simulink model "sandbox_varying"  (R2018b)
settings: Solver=VariableStepAuto  StartTime=0.0  StopTime=20  MaxStep=5e-2  RelTol=1e-3
values from neighbouring files (symbols this model uses):
  B = eye(6)    [eq_setup.m]
  G = [0, 0, m*g, 0, 0, 0]'    [eq_setup.m]
  K_E = 0.05    [eq_setup.m]
  K_m = [[ m*eye(3), zeros(3)] ... (first row only)    [eq_setup.m]
  K_p = [[  K_pt,    zeros(3)] ... (first row only)    [eq_setup.m]
  K_v = [[  K_vt,    zeros(3)] ... (first row only)    [eq_setup.m]
  M = [[ m*eye(3), zeros(3)] ... (first row only)    [eq_setup.m]
  M_inv = inv(M)    [eq_setup.m]
  xi_0 = [p_0, theta_0]    [eq_setup.m]
libraries: simulink x1
settings Model: Creator=valeriiche  LastModifiedBy=valeriiche

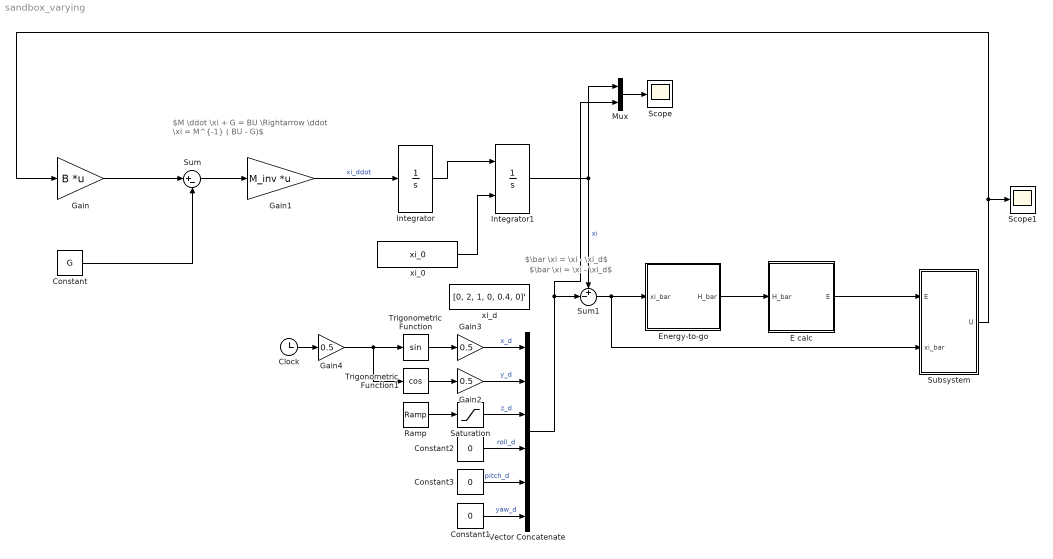
== system sandbox_varying ==
  note: $M \ddot \xi + G = BU \Rightarrow \ddot \xi = M^{-1} ( BU - G)$
  note: $\bar \xi = \xi - \xi_d$
  note: $\bar \xi = \xi - \xi_d$
  Clock : Clock
  Constant : Constant  Value=G
  Constant1 : Constant  Value=0
  Constant2 : Constant  Value=0
  Constant3 : Constant  Value=0
  E calc : Subsystem
  Energy-to-go : Subsystem
  Gain : Gain  Gain=B  Multiplication=Matrix(K*u) (u vector)
  Gain1 : Gain  Gain=M_inv  Multiplication=Matrix(K*u) (u vector)
  Gain2 : Gain  Gain=0.5
  Gain3 : Gain  Gain=0.5
  Gain4 : Gain  Gain=0.5
  Integrator : Integrator
  Integrator1 : Integrator  InitialConditionSource=external
  Mux : Mux  Inputs=2
  Ramp : simulink/Sources/Ramp  slope=0.333  start=0  InitialOutput=0
  Saturation : Saturate  UpperLimit=2  LowerLimit=0
  Scope : Scope
  Scope1 : Scope
  Subsystem : Subsystem
  Sum : Sum  Inputs=|+-
  Sum1 : Sum  Inputs=+-|
  Trigonometric Function : Trigonometry
  Trigonometric Function1 : Trigonometry  Operator=cos
  Vector Concatenate : Concatenate  NumInputs=6
  xi_0 : Constant  Value=xi_0
  xi_d : Constant  Value=[0, 2, 1, 0, 0.4, 0]'
  wires:
  Gain/1 -> Sum/1
  Constant/1 -> Sum/2
  Sum/1 -> Gain1/1
  Gain1/1 -> Integrator/1  "xi_ddot"
  Integrator/1 -> Integrator1/1
  Integrator1/1 -> Mux/1, Sum1/1  "xi"
  Sum1/1 -> Subsystem/2(xi_bar), Energy-to-go/1(xi_bar)
  E calc/1(E) -> Subsystem/1(E)
  Subsystem/1(U) -> Scope1/1, Gain/1
  xi_0/1 -> Integrator1/2
  Energy-to-go/1(H_bar) -> E calc/1(H_bar)
  Vector Concatenate/1 -> Mux/2, Sum1/2
  Constant2/1 -> Vector Concatenate/4  "roll_d"
  Constant3/1 -> Vector Concatenate/5  "pitch_d"
  Saturation/1 -> Vector Concatenate/3  "z_d"
  Ramp/1 -> Saturation/1
  Gain2/1 -> Vector Concatenate/2  "y_d"
  Trigonometric Function1/1 -> Gain2/1
  Gain3/1 -> Vector Concatenate/1  "x_d"
  Trigonometric Function/1 -> Gain3/1
  Clock/1 -> Gain4/1
  Gain4/1 -> Trigonometric Function1/1, Trigonometric Function/1
  Constant1/1 -> Vector Concatenate/6  "yaw_d"
  Mux/1 -> Scope/1

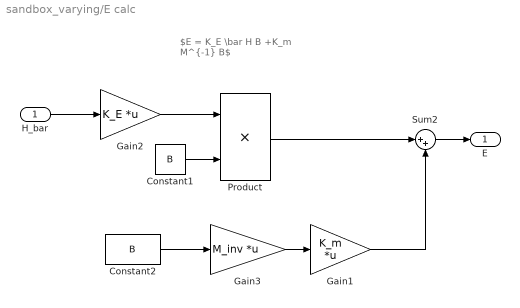
== system sandbox_varying/E calc ==
  note: $E = K_E \bar H B +K_m M^{-1} B$
  H_bar : Inport
  Constant1 : Constant  Value=B
  Constant2 : Constant  Value=B
  Gain1 : Gain  Gain=K_m  Multiplication=Matrix(K*u)
  Gain2 : Gain  Gain=K_E  Multiplication=Matrix(K*u) (u vector)
  Gain3 : Gain  Gain=M_inv  Multiplication=Matrix(K*u)
  Product : Product
  Sum2 : Sum  Inputs=|++
  E : Outport
  wires:
  Constant1/1 -> Product/2
  H_bar/1 -> Gain2/1
  Constant2/1 -> Gain3/1
  Sum2/1 -> E/1
  Gain2/1 -> Product/1
  Product/1 -> Sum2/1
  Gain3/1 -> Gain1/1
  Gain1/1 -> Sum2/2

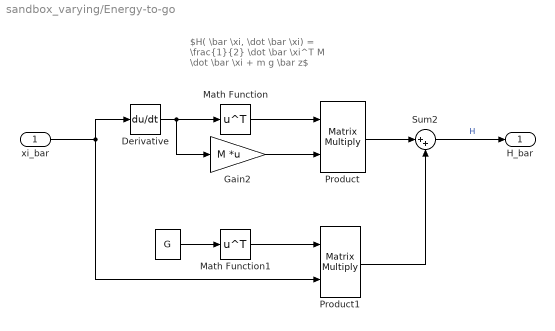
== system sandbox_varying/Energy-to-go ==
  note: $H( \bar \xi, \dot \bar \xi) = \frac{1}{2} \dot \bar \xi^T M \dot \bar \xi + m g \bar z$
  xi_bar : Inport
  " " : Constant  Value=G
  Derivative : Derivative
  Gain2 : Gain  Gain=M  Multiplication=Matrix(K*u) (u vector)
  Math Function : Math  Operator=transpose  SaturateOnIntegerOverflow=on
  Math Function1 : Math  Operator=transpose  SaturateOnIntegerOverflow=on
  Product : Product  Multiplication=Matrix(*)
  Product1 : Product  Multiplication=Matrix(*)
  Sum2 : Sum  Inputs=|++
  H_bar : Outport
  wires:
  Sum2/1 -> H_bar/1  "H"
  xi_bar/1 -> Product1/2, Derivative/1
  Derivative/1 -> Gain2/1, Math Function/1
  Product1/1 -> Sum2/2
  Product/1 -> Sum2/1
  Gain2/1 -> Product/2
  Math Function/1 -> Product/1
  Math Function1/1 -> Product1/1
  " "/1 -> Math Function1/1

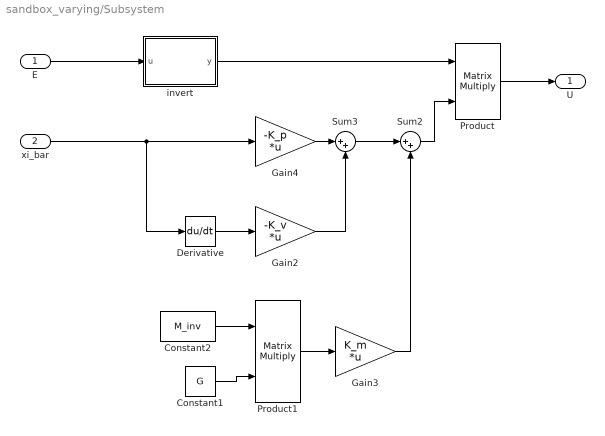
== system sandbox_varying/Subsystem ==
  E : Inport
  xi_bar : Inport  Port=2
  Constant1 : Constant  Value=G
  Constant2 : Constant  Value=M_inv
  Derivative : Derivative
  Gain2 : Gain  Gain=-K_v  Multiplication=Matrix(K*u) (u vector)
  Gain3 : Gain  Gain=K_m  Multiplication=Matrix(K*u)
  Gain4 : Gain  Gain=-K_p  Multiplication=Matrix(K*u) (u vector)
  Product : Product  Multiplication=Matrix(*)
  Product1 : Product  Multiplication=Matrix(*)
  Sum2 : Sum  Inputs=|++
  Sum3 : Sum  Inputs=|++
  invert : MATLAB Function  TreatAsAtomicUnit=on
  U : Outport
  wires:
  Derivative/1 -> Gain2/1
  Gain2/1 -> Sum3/2
  Product/1 -> U/1
  invert/1(y) -> Product/1
  Sum3/1 -> Sum2/1
  Gain4/1 -> Sum3/1
  Constant1/1 -> Product1/2
  Sum2/1 -> Product/2
  E/1 -> invert/1(u)
  xi_bar/1 -> Derivative/1, Gain4/1
  Constant2/1 -> Product1/1
  Product1/1 -> Gain3/1
  Gain3/1 -> Sum2/2

== matlab function sandbox_varying/Subsystem/invert ==
  data: u input; y output
function y = fcn(u)
    
y = inv(u);
